simulink model "compound_pendulum"  (R2019b)
settings: Solver=VariableStepAuto  StartTime=0.0  StopTime=80  RelTol=1e-3
undefined symbols (not defined in the file): c, d, g, J, L, m
libraries: simulink_extras x2, fuzblock x1
settings Model: Creator=guess  LastModifiedBy=guess
settings SolverCC: ZeroCrossControl=DisableAll
settings OptimizationCC: BooleanDataType=off

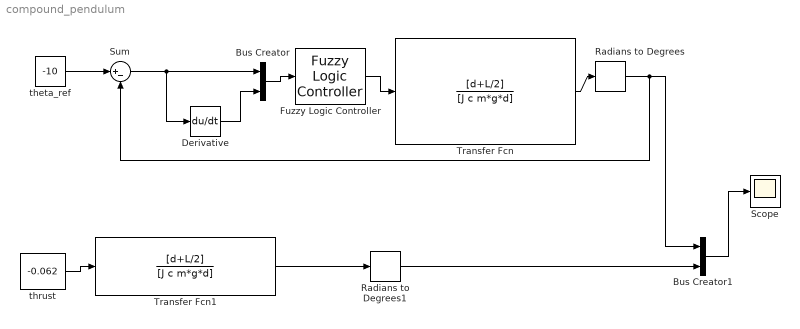
== system compound_pendulum ==
  Bus Creator : BusCreator  Inputs=2
  Bus Creator1 : BusCreator  Inputs=2
  Derivative : Derivative
  Fuzzy Logic Controller : fuzblock/Fuzzy Logic  Controller  FIS=CompoundPendulum  OutputSampleNumber=101  DataType=double  FuzzifiedInputs=off  RuleFiringStrengths=off  RuleOutputs=off  AggregatedOutputs=off  SimulateUsing=Interpreted execution  OutOfRangeInputValueMessage=warning  NoRuleFiredMessage=warning  EmptyOutputFuzzySetMessage=warning
  Radians to Degrees : simulink_extras/Transformations/Radians to Degrees
  Radians to Degrees1 : simulink_extras/Transformations/Radians to Degrees
  Scope : Scope
  Sum : Sum  Inputs=|+-
  Transfer Fcn : TransferFcn  Numerator=[d+L/2]  Denominator=[J c m*g*d]
  Transfer Fcn1 : TransferFcn  Numerator=[d+L/2]  Denominator=[J c m*g*d]
  theta_ref : Constant  Value=-10
  thrust : Constant  Value=-0.062
  wires:
  Sum/1 -> Bus Creator/1, Derivative/1
  theta_ref/1 -> Sum/1
  thrust/1 -> Transfer Fcn1/1
  Bus Creator/1 -> Fuzzy Logic Controller/1
  Derivative/1 -> Bus Creator/2
  Fuzzy Logic Controller/1 -> Transfer Fcn/1
  Transfer Fcn/1 -> Radians to Degrees/1
  Radians to Degrees/1 -> Sum/2, Bus Creator1/1
  Bus Creator1/1 -> Scope/1
  Radians to Degrees1/1 -> Bus Creator1/2
  Transfer Fcn1/1 -> Radians to Degrees1/1
